simulink model "generic_Truck_And_Trailer"  (R2025a)
settings: Solver=VariableStepAuto  StartTime=0.0  StopTime=350  FixedStep=0.01  MaxStep=0.001  RelTol=1e-3  EnableMultiTasking=on
libraries: TruckMaker4SL x250, simulink x1
(part 4 of 11)

== system generic_Truck_And_Trailer/TruckMaker/Tractor_Subsystem /Subsystem_Noisey Measurements/Measurements from IMU ==
  Acc_x : TruckMaker4SL/Read CM Dict  xname=Sensor.Inertial.Vhcl.VchBdy.Acc_B.x  xsync=off  xstime=Continuous
      settings: SourceProductName=TruckMaker4SL
  Acc_y : TruckMaker4SL/Read CM Dict  xname=Sensor.Inertial.Vhcl.VchBdy.Acc_B.y  xsync=off  xstime=Continuous
      settings: SourceProductName=TruckMaker4SL
  Acc_z : TruckMaker4SL/Read CM Dict  xname=Sensor.Inertial.Vhcl.VchBdy.Acc_B.z  xsync=off  xstime=Continuous
      settings: SourceProductName=TruckMaker4SL
  Omega_z : TruckMaker4SL/Read CM Dict  xname=Sensor.Inertial.Vhcl.VchBdy.Omega_B.z  xsync=off  xstime=Continuous
      settings: SourceProductName=TruckMaker4SL
  Omega_z1 : TruckMaker4SL/Read CM Dict  xname=Sensor.Inertial.Vhcl.VchBdy.Omega_B.y  xsync=off  xstime=Continuous
      settings: SourceProductName=TruckMaker4SL
  Omega_z2 : TruckMaker4SL/Read CM Dict  xname=Sensor.Inertial.Vhcl.VchBdy.Omega_B.x  xsync=off  xstime=Continuous
      settings: SourceProductName=TruckMaker4SL
  Vel_x : TruckMaker4SL/Read CM Dict  xname=Sensor.Inertial.Vhcl.VchBdy.Vel_B.x  xsync=off  xstime=Continuous
      settings: SourceProductName=TruckMaker4SL
  Vel_y : TruckMaker4SL/Read CM Dict  xname=Sensor.Inertial.Vhcl.VchBdy.Vel_B.y  xsync=off  xstime=Continuous
      settings: SourceProductName=TruckMaker4SL
  Vel_z : TruckMaker4SL/Read CM Dict  xname=Sensor.Inertial.Vhcl.VchBdy.Vel_B.z  xsync=off  xstime=Continuous
      settings: SourceProductName=TruckMaker4SL
  acc_x : Outport
  acc_y : Outport  Port=2
  acc_z : Outport  Port=3
  vel_x : Outport  Port=4
  vel_y : Outport  Port=5
  vel_z : Outport  Port=6
  wx : Outport  Port=7
  wy : Outport  Port=8
  wz : Outport  Port=9
  wires:
  Omega_z/1 -> wz/1
  Omega_z1/1 -> wy/1
  Omega_z2/1 -> wx/1
  Vel_z/1 -> vel_z/1
  Vel_y/1 -> vel_y/1
  Vel_x/1 -> vel_x/1
  Acc_z/1 -> acc_z/1
  Acc_y/1 -> acc_y/1
  Acc_x/1 -> acc_x/1

== system generic_Truck_And_Trailer/TruckMaker/Tractor_Subsystem /Subsystem_Noisey Measurements _NAN/Measurements from IMU ==
  Acc_x : TruckMaker4SL/Read CM Dict  xname=Sensor.Inertial.Vhcl.VchBdy.Acc_B.x  xsync=off  xstime=Continuous
      settings: SourceProductName=TruckMaker4SL
  Acc_y : TruckMaker4SL/Read CM Dict  xname=Sensor.Inertial.Vhcl.VchBdy.Acc_B.y  xsync=off  xstime=Continuous
      settings: SourceProductName=TruckMaker4SL
  Acc_z : TruckMaker4SL/Read CM Dict  xname=Sensor.Inertial.Vhcl.VchBdy.Acc_B.z  xsync=off  xstime=Continuous
      settings: SourceProductName=TruckMaker4SL
  Omega_z : TruckMaker4SL/Read CM Dict  xname=Sensor.Inertial.Vhcl.VchBdy.Omega_B.z  xsync=off  xstime=Continuous
      settings: SourceProductName=TruckMaker4SL
  Omega_z1 : TruckMaker4SL/Read CM Dict  xname=Sensor.Inertial.Vhcl.VchBdy.Omega_B.y  xsync=off  xstime=Continuous
      settings: SourceProductName=TruckMaker4SL
  Omega_z2 : TruckMaker4SL/Read CM Dict  xname=Sensor.Inertial.Vhcl.VchBdy.Omega_B.x  xsync=off  xstime=Continuous
      settings: SourceProductName=TruckMaker4SL
  Vel_x : TruckMaker4SL/Read CM Dict  xname=Sensor.Inertial.Vhcl.VchBdy.Vel_B.x  xsync=off  xstime=Continuous
      settings: SourceProductName=TruckMaker4SL
  Vel_y : TruckMaker4SL/Read CM Dict  xname=Sensor.Inertial.Vhcl.VchBdy.Vel_B.y  xsync=off  xstime=Continuous
      settings: SourceProductName=TruckMaker4SL
  Vel_z : TruckMaker4SL/Read CM Dict  xname=Sensor.Inertial.Vhcl.VchBdy.Vel_B.z  xsync=off  xstime=Continuous
      settings: SourceProductName=TruckMaker4SL
  acc_x : Outport
  acc_y : Outport  Port=2
  acc_z : Outport  Port=3
  vel_x : Outport  Port=4
  vel_y : Outport  Port=5
  vel_z : Outport  Port=6
  wx : Outport  Port=7
  wy : Outport  Port=8
  wz : Outport  Port=9
  wires:
  Acc_x/1 -> acc_x/1
  Acc_y/1 -> acc_y/1
  Acc_z/1 -> acc_z/1
  Vel_x/1 -> vel_x/1
  Vel_y/1 -> vel_y/1
  Vel_z/1 -> vel_z/1
  Omega_z2/1 -> wx/1
  Omega_z1/1 -> wy/1
  Omega_z/1 -> wz/1

== system generic_Truck_And_Trailer/TruckMaker/IPG Vehicle/CarAndTrailer/CarAndTrailerUpd/CreateBus Brake.IF.In ==
  In : Inport
  BusCreator : BusCreator  Inputs=25
  Demux : Demux  Outputs=25
      settings: DisplayOption=none
  Out : Outport  VectorParamsAs1DForOutWhenUnconnected=off
  wires:
  Demux/25 -> BusCreator/25  "Brake IF Trq_Reg RR4"
  Demux/24 -> BusCreator/24  "Brake IF Trq_Reg RL4"
  Demux/23 -> BusCreator/23  "Brake IF Trq_Reg RR3"
  Demux/22 -> BusCreator/22  "Brake IF Trq_Reg RL3"
  Demux/21 -> BusCreator/21  "Brake IF Trq_Reg FR2"
  Demux/20 -> BusCreator/20  "Brake IF Trq_Reg FL2"
  Demux/19 -> BusCreator/19  "Brake IF Trq_Reg RR2"
  Demux/18 -> BusCreator/18  "Brake IF Trq_Reg RL2"
  Demux/17 -> BusCreator/17  "Brake IF Trq_Reg RR"
  Demux/16 -> BusCreator/16  "Brake IF Trq_Reg RL"
  Demux/15 -> BusCreator/15  "Brake IF Trq_Reg FR"
  Demux/14 -> BusCreator/14  "Brake IF Trq_Reg FL"
  Demux/13 -> BusCreator/13  "Brake IF Trq_Reg_max RR4"
  Demux/12 -> BusCreator/12  "Brake IF Trq_Reg_max RL4"
  Demux/11 -> BusCreator/11  "Brake IF Trq_Reg_max RR3"
  Demux/10 -> BusCreator/10  "Brake IF Trq_Reg_max RL3"
  Demux/9 -> BusCreator/9  "Brake IF Trq_Reg_max FR2"
  Demux/8 -> BusCreator/8  "Brake IF Trq_Reg_max FL2"
  Demux/7 -> BusCreator/7  "Brake IF Trq_Reg_max RR2"
  Demux/6 -> BusCreator/6  "Brake IF Trq_Reg_max RL2"
  Demux/5 -> BusCreator/5  "Brake IF Trq_Reg_max RR"
  Demux/4 -> BusCreator/4  "Brake IF Trq_Reg_max RL"
  Demux/3 -> BusCreator/3  "Brake IF Trq_Reg_max FR"
  Demux/2 -> BusCreator/2  "Brake IF Trq_Reg_max FL"
  Demux/1 -> BusCreator/1  "Brake IF T_env"
  BusCreator/1 -> Out/1
  In/1 -> Demux/1

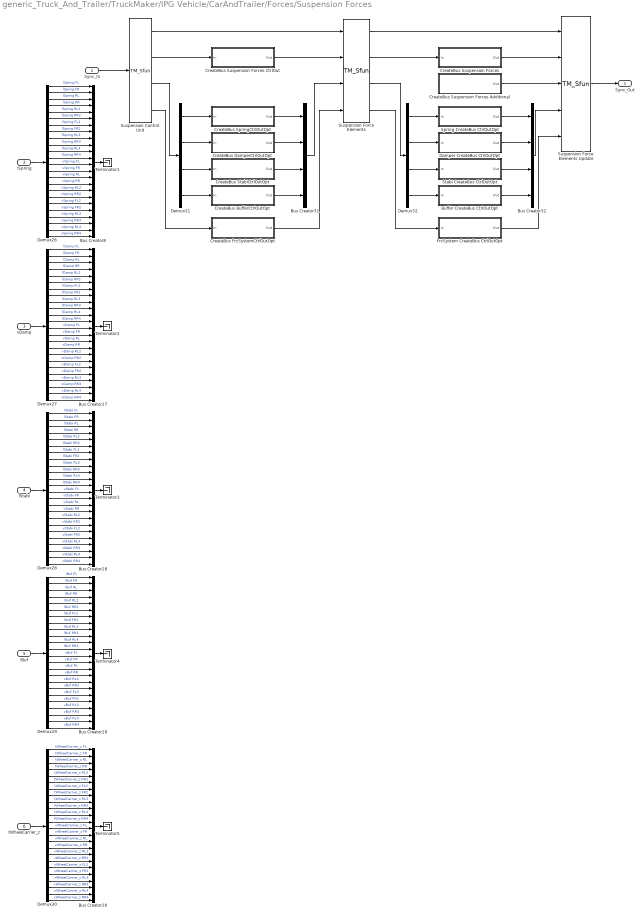
== system generic_Truck_And_Trailer/TruckMaker/IPG Vehicle/CarAndTrailer/Forces/Suspension Forces ==
  Sync_In : Inport
  lSpring : Inport  Port=2
  vDamp : Inport  Port=3
  lStabi : Inport  Port=4
  lBuf : Inport  Port=5
  tWheelCarrier_z : Inport  Port=6
  Buffer CreateBus CtrlOutOpt : Subsystem
  Bus Creator{8,27..30} (5 alike) : BusCreator  Inputs=24
  Bus Creator31 : BusCreator  Inputs=4
  Bus Creator32 : BusCreator  Inputs=4
  CreateBus BufferCtrlOutOpt : Subsystem
  CreateBus DamperCtrlOutOpt : Subsystem
  CreateBus FrcSystemCtrlOutOpt : Subsystem
  CreateBus SpringCtrlOutOpt : Subsystem
  CreateBus StabiCtrlOutOpt : Subsystem
  CreateBus Suspension Forces : Subsystem
  CreateBus Suspension Forces Additional : Subsystem
  CreateBus Suspension Forces CtrlOut : Subsystem
  Damper CreateBus CtrlOutOpt : Subsystem
  Demux{26..30} (5 alike) : Demux  Outputs=24
      settings: DisplayOption=none
  Demux31 : Demux
      settings: DisplayOption=none
  Demux32 : Demux
      settings: DisplayOption=none
  FrcSystem CreateBus CtrlOutOpt : Subsystem
  Spring CreateBus CtrlOutOpt : Subsystem
  Stabi CreateBus CtrlOutOpt : Subsystem
  Suspension Control Unit : S-Function  FunctionName=TM_Sfun  Parameters='ForcesSuspControl'  SFunctionDeploymentMode=off  EnableBusSupport=off
  Suspension Force Elements : S-Function  FunctionName=TM_Sfun  Parameters='ForcesSusp'  SFunctionDeploymentMode=off  EnableBusSupport=off
  Suspension Force Elements Update : S-Function  FunctionName=TM_Sfun  Parameters='ForcesSuspUpd'  SFunctionDeploymentMode=off  EnableBusSupport=off
  Terminator{1..5} (5 alike) : Terminator
  Sync_Out : Outport  VectorParamsAs1DForOutWhenUnconnected=off
  wires:
  CreateBus Suspension Forces CtrlOut/1(Out) -> Suspension Force Elements/2
  Suspension Control Unit/2 -> CreateBus Suspension Forces CtrlOut/1(In)
  Suspension Force Elements Update/1 -> Sync_Out/1
  Suspension Force Elements/1 -> Suspension Force Elements Update/1
  Suspension Control Unit/1 -> Suspension Force Elements/1
  Sync_In/1 -> Suspension Control Unit/1
  CreateBus Suspension Forces Additional/1(Out) -> Suspension Force Elements Update/3
  Demux27/20 -> Bus Creator27/20  "vDamp FR2"
  Demux29/8 -> Bus Creator29/8  "lBuf FR2"
  Demux27/10 -> Bus Creator27/10  "lDamp RR3"
  Demux29/12 -> Bus Creator29/12  "lBuf RR4"
  Demux26/21 -> Bus Creator8/21  "vSpring RL3"
  Demux29/11 -> Bus Creator29/11  "lBuf RL4"
  Demux26/5 -> Bus Creator8/5  "lSpring RL2"
  Demux27/23 -> Bus Creator27/23  "vDamp RL4"
  Demux27/7 -> Bus Creator27/7  "lDamp FL2"
  Demux29/17 -> Bus Creator29/17  "vBuf RL2"
  lBuf/1 -> Demux29/1
  Demux27/21 -> Bus Creator27/21  "vDamp RL3"
  Demux26/17 -> Bus Creator8/17  "vSpring RL2"
  Demux28/17 -> Bus Creator28/17  "vStabi RL2"
  Demux27/6 -> Bus Creator27/6  "lDamp RR2"
  Demux26/16 -> Bus Creator8/16  "vSpring RR"
  vDamp/1 -> Demux27/1
  Demux28/13 -> Bus Creator28/13  "vStabi FL"
  Demux27/3 -> Bus Creator27/3  "lDamp RL"
  Demux28/24 -> Bus Creator28/24  "vStabi RR4"
  Demux29/9 -> Bus Creator29/9  "lBuf RL3"
  Demux27/17 -> Bus Creator27/17  "vDamp RL2"
  Demux28/9 -> Bus Creator28/9  "lStabi RL3"
  Demux29/5 -> Bus Creator29/5  "lBuf RL2"
  Demux28/12 -> Bus Creator28/12  "lStabi RR4"
  Demux26/12 -> Bus Creator8/12  "lSpring RR4"
  Demux26/24 -> Bus Creator8/24  "vSpring RR4"
  Demux28/23 -> Bus Creator28/23  "vStabi RL4"
  Demux26/4 -> Bus Creator8/4  "lSpring RR"
  Demux28/4 -> Bus Creator28/4  "lStabi RR"
  Demux29/3 -> Bus Creator29/3  "lBuf RL"
  Demux28/14 -> Bus Creator28/14  "vStabi FR"
  Demux27/12 -> Bus Creator27/12  "lDamp RR4"
  Demux28/8 -> Bus Creator28/8  "lStabi FR2"
  Demux29/6 -> Bus Creator29/6  "lBuf RR2"
  Demux27/14 -> Bus Creator27/14  "vDamp FR"
  Bus Creator29/1 -> Terminator4/1
  Demux28/7 -> Bus Creator28/7  "lStabi FL2"
  Demux29/1 -> Bus Creator29/1  "lBuf FL"
  Demux27/2 -> Bus Creator27/2  "lDamp FR"
  Demux26/9 -> Bus Creator8/9  "lSpring RL3"
  Demux26/7 -> Bus Creator8/7  "lSpring FL2"
  Demux29/4 -> Bus Creator29/4  "lBuf RR"
  Demux28/11 -> Bus Creator28/11  "lStabi RL4"
  Demux28/10 -> Bus Creator28/10  "lStabi RR3"
  Demux28/1 -> Bus Creator28/1  "lStabi FL"
  lStabi/1 -> Demux28/1
  Demux26/14 -> Bus Creator8/14  "vSpring FR"
  Demux28/21 -> Bus Creator28/21  "vStabi RL3"
  Demux26/15 -> Bus Creator8/15  "vSpring RL"
  Demux28/2 -> Bus Creator28/2  "lStabi FR"
  Demux28/15 -> Bus Creator28/15  "vStabi RL"
  Demux28/19 -> Bus Creator28/19  "vStabi FL2"
  Demux28/16 -> Bus Creator28/16  "vStabi RR"
  Demux28/6 -> Bus Creator28/6  "lStabi RR2"
  Demux29/22 -> Bus Creator29/22  "vBuf RR3"
  Demux27/15 -> Bus Creator27/15  "vDamp RL"
  Demux27/5 -> Bus Creator27/5  "lDamp RL2"
  Demux29/15 -> Bus Creator29/15  "vBuf RL"
  Demux29/13 -> Bus Creator29/13  "vBuf FL"
  Demux26/13 -> Bus Creator8/13  "vSpring FL"
  Demux27/1 -> Bus Creator27/1  "lDamp FL"
  Demux26/18 -> Bus Creator8/18  "vSpring RR2"
  Demux28/5 -> Bus Creator28/5  "lStabi RL2"
  Demux29/10 -> Bus Creator29/10  "lBuf RR3"
  Demux28/18 -> Bus Creator28/18  "vStabi RR2"
  Demux27/11 -> Bus Creator27/11  "lDamp RL4"
  Demux27/9 -> Bus Creator27/9  "lDamp RL3"
  Demux27/18 -> Bus Creator27/18  "vDamp RR2"
  Demux29/16 -> Bus Creator29/16  "vBuf RR"
  Demux27/8 -> Bus Creator27/8  "lDamp FR2"
  Demux26/2 -> Bus Creator8/2  "lSpring FR"
  Demux26/1 -> Bus Creator8/1  "lSpring FL"
  Demux29/24 -> Bus Creator29/24  "vBuf RR4"
  Demux27/19 -> Bus Creator27/19  "vDamp FL2"
  Demux29/2 -> Bus Creator29/2  "lBuf FR"
  Demux27/24 -> Bus Creator27/24  "vDamp RR4"
  Demux27/4 -> Bus Creator27/4  "lDamp RR"
  Demux26/3 -> Bus Creator8/3  "lSpring RL"
  Demux28/20 -> Bus Creator28/20  "vStabi FR2"
  Demux26/6 -> Bus Creator8/6  "lSpring RR2"
  Demux29/14 -> Bus Creator29/14  "vBuf FR"
  Demux27/16 -> Bus Creator27/16  "vDamp RR"
  Demux27/22 -> Bus Creator27/22  "vDamp RR3"
  lSpring/1 -> Demux26/1
  Demux26/11 -> Bus Creator8/11  "lSpring RL4"
  Demux26/22 -> Bus Creator8/22  "vSpring RR3"
  Bus Creator27/1 -> Terminator2/1
  Demux29/18 -> Bus Creator29/18  "vBuf RR2"
  Demux26/10 -> Bus Creator8/10  "lSpring RR3"
  Bus Creator28/1 -> Terminator3/1
  Demux26/8 -> Bus Creator8/8  "lSpring FR2"
  Demux26/19 -> Bus Creator8/19  "vSpring FL2"
  Bus Creator8/1 -> Terminator1/1
  Demux29/23 -> Bus Creator29/23  "vBuf RL4"
  Demux29/21 -> Bus Creator29/21  "vBuf RL3"
  Demux26/23 -> Bus Creator8/23  "vSpring RL4"
  Demux29/19 -> Bus Creator29/19  "vBuf FL2"
  Demux28/22 -> Bus Creator28/22  "vStabi RR3"
  Demux28/3 -> Bus Creator28/3  "lStabi RL"
  Demux27/13 -> Bus Creator27/13  "vDamp FL"
  Demux29/7 -> Bus Creator29/7  "lBuf FL2"
  Demux26/20 -> Bus Creator8/20  "vSpring FR2"
  Demux29/20 -> Bus Creator29/20  "vBuf FR2"
  Demux30/15 -> Bus Creator30/15  "vWheelCarrier_z RL"
  Demux30/11 -> Bus Creator30/11  "tWheelCarrier_z RL4"
  Demux30/16 -> Bus Creator30/16  "vWheelCarrier_z RR"
  Demux30/24 -> Bus Creator30/24  "vWheelCarrier_z RR4"
  Demux30/8 -> Bus Creator30/8  "tWheelCarrier_z FR2"
  Demux30/18 -> Bus Creator30/18  "vWheelCarrier_z RR2"
  Demux30/9 -> Bus Creator30/9  "tWheelCarrier_z RL3"
  Demux30/22 -> Bus Creator30/22  "vWheelCarrier_z RR3"
  Demux30/3 -> Bus Creator30/3  "tWheelCarrier_z RL"
  Bus Creator30/1 -> Terminator5/1
  Demux30/7 -> Bus Creator30/7  "tWheelCarrier_z FL2"
  Demux30/5 -> Bus Creator30/5  "tWheelCarrier_z RL2"
  Demux30/21 -> Bus Creator30/21  "vWheelCarrier_z RL3"
  Demux30/10 -> Bus Creator30/10  "tWheelCarrier_z RR3"
  Demux30/2 -> Bus Creator30/2  "tWheelCarrier_z FR"
  Demux30/19 -> Bus Creator30/19  "vWheelCarrier_z FL2"
  Demux30/4 -> Bus Creator30/4  "tWheelCarrier_z RR"
  Demux30/23 -> Bus Creator30/23  "vWheelCarrier_z RL4"
  Demux30/13 -> Bus Creator30/13  "vWheelCarrier_z FL"
  Demux30/17 -> Bus Creator30/17  "vWheelCarrier_z RL2"
  Demux30/14 -> Bus Creator30/14  "vWheelCarrier_z FR"
  Demux30/6 -> Bus Creator30/6  "tWheelCarrier_z RR2"
  Demux30/20 -> Bus Creator30/20  "vWheelCarrier_z FR2"
  tWheelCarrier_z/1 -> Demux30/1
  Demux30/12 -> Bus Creator30/12  "tWheelCarrier_z RR4"
  Demux30/1 -> Bus Creator30/1  "tWheelCarrier_z FL"
  CreateBus DamperCtrlOutOpt/1(Out) -> Bus Creator31/2
  CreateBus StabiCtrlOutOpt/1(Out) -> Bus Creator31/3
  Suspension Control Unit/4 -> CreateBus FrcSystemCtrlOutOpt/1(In)
  CreateBus SpringCtrlOutOpt/1(Out) -> Bus Creator31/1
  Demux31/3 -> CreateBus StabiCtrlOutOpt/1(In)
  Demux31/2 -> CreateBus DamperCtrlOutOpt/1(In)
  Demux31/1 -> CreateBus SpringCtrlOutOpt/1(In)
  CreateBus FrcSystemCtrlOutOpt/1(Out) -> Suspension Force Elements/4
  Demux31/4 -> CreateBus BufferCtrlOutOpt/1(In)
  CreateBus BufferCtrlOutOpt/1(Out) -> Bus Creator31/4
  Suspension Control Unit/3 -> Demux31/1
  Bus Creator31/1 -> Suspension Force Elements/3
  Spring CreateBus CtrlOutOpt/1(Out) -> Bus Creator32/1
  Demux32/2 -> Damper CreateBus CtrlOutOpt/1(In)
  Damper CreateBus CtrlOutOpt/1(Out) -> Bus Creator32/2
  Buffer CreateBus CtrlOutOpt/1(Out) -> Bus Creator32/4
  Demux32/4 -> Buffer CreateBus CtrlOutOpt/1(In)
  Demux32/1 -> Spring CreateBus CtrlOutOpt/1(In)
  Stabi CreateBus CtrlOutOpt/1(Out) -> Bus Creator32/3
  Demux32/3 -> Stabi CreateBus CtrlOutOpt/1(In)
  Suspension Force Elements/2 -> CreateBus Suspension Forces/1(In)
  CreateBus Suspension Forces/1(Out) -> Suspension Force Elements Update/2
  Suspension Force Elements/3 -> Demux32/1
  Suspension Force Elements/4 -> FrcSystem CreateBus CtrlOutOpt/1(In)
  Bus Creator32/1 -> Suspension Force Elements Update/4
  FrcSystem CreateBus CtrlOutOpt/1(Out) -> Suspension Force Elements Update/5

== system generic_Truck_And_Trailer/TruckMaker/IPG Vehicle/CarAndTrailer/Forces/Vehicle Forces ==
  Sync_In : Inport
  Bus Creator1 : BusCreator  Inputs=12
  Bus Creator8 : BusCreator  Inputs=16
  BusCreator1 : BusCreator  Inputs=4
  BusCreator2 : BusCreator  Inputs=9
  Demux : Demux  Outputs=16
      settings: DisplayOption=none
  Demux1 : Demux  Outputs=12
      settings: DisplayOption=none
  Demux2 : Demux  Outputs=13
      settings: DisplayOption=none
  Forces : S-Function  FunctionName=TM_Sfun  Parameters='Forces'  SFunctionDeploymentMode=off  EnableBusSupport=off
  Terminator : Terminator
  Sync_Out : Outport  VectorParamsAs1DForOutWhenUnconnected=off
  Car.Virtual : Outport  Port=2  VectorParamsAs1DForOutWhenUnconnected=off
  Car.Aero : Outport  Port=3  VectorParamsAs1DForOutWhenUnconnected=off
  Car.Load : Outport  Port=4  VectorParamsAs1DForOutWhenUnconnected=off
  wires:
  BusCreator1/1 -> Terminator/1  "Aero IF (in)"
  Demux2/13 -> BusCreator2/9  "car Aero Trq_1 z"
  Demux2/12 -> BusCreator2/8  "car Aero Trq_1 y"
  Demux2/11 -> BusCreator2/7  "car Aero Trq_1 x"
  Demux2/10 -> BusCreator2/6  "car Aero Frc_1 z"
  Demux2/9 -> BusCreator2/5  "car Aero Frc_1 y"
  Demux2/8 -> BusCreator2/4  "car Aero Frc_1 x"
  Demux2/7 -> BusCreator2/3  "car Aero PoA_1 z"
  Demux2/6 -> BusCreator2/2  "car Aero PoA_1 y"
  Demux2/5 -> BusCreator2/1  "car Aero PoA_1 x"
  Demux2/4 -> BusCreator1/4  "car Aero tau_1"
  Demux2/3 -> BusCreator1/3  "car Aero ApproachVel_1 z"
  Demux2/2 -> BusCreator1/2  "car Aero ApproachVel_1 y"
  Demux2/1 -> BusCreator1/1  "car Aero ApproachVel_1 x"
  BusCreator2/1 -> Car.Aero/1
  Demux/16 -> Bus Creator8/16  "Car Load_3 tz"
  Demux/15 -> Bus Creator8/15  "Car Load_3 ty"
  Demux/14 -> Bus Creator8/14  "Car Load_3 tx"
  Demux/13 -> Bus Creator8/13  "Car Load_3 mass"
  Demux1/12 -> Bus Creator1/12  "Car Virtual Trq_0 z"
  Demux1/11 -> Bus Creator1/11  "Car Virtual Trq_0 y"
  Demux1/10 -> Bus Creator1/10  "Car Virtual Trq_0 x"
  Demux1/9 -> Bus Creator1/9  "Car Virtual Trq_1 z"
  Demux1/8 -> Bus Creator1/8  "Car Virtual Trq_1 y"
  Demux1/7 -> Bus Creator1/7  "Car Virtual Trq_1 x"
  Demux1/6 -> Bus Creator1/6  "Car Virtual Frc_0 z"
  Demux1/5 -> Bus Creator1/5  "Car Virtual Frc_0 y"
  Demux1/4 -> Bus Creator1/4  "Car Virtual Frc_0 x"
  Sync_In/1 -> Forces/1
  Forces/1 -> Sync_Out/1
  Demux1/1 -> Bus Creator1/1  "Car Virtual Frc_1 x"
  Demux1/2 -> Bus Creator1/2  "Car Virtual Frc_1 y"
  Demux1/3 -> Bus Creator1/3  "Car Virtual Frc_1 z"
  Forces/3 -> Demux2/1
  Forces/2 -> Demux1/1
  Bus Creator1/1 -> Car.Virtual/1
  Bus Creator8/1 -> Car.Load/1
  Demux/1 -> Bus Creator8/1  "Car Load_0 mass"
  Demux/2 -> Bus Creator8/2  "Car Load_0 tx"
  Demux/3 -> Bus Creator8/3  "Car Load_0 ty"
  Demux/4 -> Bus Creator8/4  "Car Load_0 tz"
  Demux/5 -> Bus Creator8/5  "Car Load_1 mass"
  Demux/6 -> Bus Creator8/6  "Car Load_1 tx"
  Demux/7 -> Bus Creator8/7  "Car Load_1 ty"
  Demux/8 -> Bus Creator8/8  "Car Load_1 tz"
  Demux/9 -> Bus Creator8/9  "Car Load_2 mass"
  Demux/10 -> Bus Creator8/10  "Car Load_2 tx"
  Demux/11 -> Bus Creator8/11  "Car Load_2 ty"
  Demux/12 -> Bus Creator8/12  "Car Load_2 tz"
  Forces/4 -> Demux/1

== system generic_Truck_And_Trailer/TruckMaker/IPG Vehicle/CarAndTrailer/Trailer/CreateBus Car.Hitch.FrcTrq ==
  In1 : Inport
  Bus Creator7 : BusCreator  Inputs=6
  Demux7 : Demux  Outputs=6
      settings: DisplayOption=none
  Out1 : Outport  VectorParamsAs1DForOutWhenUnconnected=off
  wires:
  In1/1 -> Demux7/1
  Bus Creator7/1 -> Out1/1
  Demux7/6 -> Bus Creator7/6  "Car Hitch Trq2Car z"
  Demux7/5 -> Bus Creator7/5  "Car Hitch Trq2Car y"
  Demux7/4 -> Bus Creator7/4  "Car Hitch Trq2Car x"
  Demux7/3 -> Bus Creator7/3  "Car Hitch Frc2Car z"
  Demux7/2 -> Bus Creator7/2  "Car Hitch Frc2Car y"
  Demux7/1 -> Bus Creator7/1  "Car Hitch Frc2Car x"

== system generic_Truck_And_Trailer/TruckMaker/IPG Vehicle/CarAndTrailer/Trailer/CreateBus Vhcl.Motion ==
  In1 : Inport
  BusCreator : BusCreator  Inputs=15
  Demux : Demux  Outputs=15
      settings: DisplayOption=none
  Mux : Mux  Inputs=2
  Scope : Scope
      settings: ActiveDisplayYMinimum=-2.4357036031707069  ActiveDisplayYMaximum=21.91421659683628  DataLoggingVariableName=ScopeData2
  Out1 : Outport  VectorParamsAs1DForOutWhenUnconnected=off
  wires:
  Demux/15 -> BusCreator/15  "Vhcl YawAcc"
  Demux/14 -> Mux/2, BusCreator/14  "Vhcl YawVel"
  Demux/13 -> BusCreator/13  "Vhcl Yaw"
  Demux/12 -> BusCreator/12  "Vhcl PitchAcc"
  Demux/11 -> BusCreator/11  "Vhcl PitchVel"
  Demux/10 -> BusCreator/10  "Vhcl Pitch"
  Demux/9 -> BusCreator/9  "Vhcl RollAcc"
  Demux/8 -> BusCreator/8  "Vhcl RollVel"
  Demux/7 -> BusCreator/7  "Vhcl Roll"
  Demux/6 -> BusCreator/6  "Vhcl Hitch_Pos z"
  Demux/5 -> BusCreator/5  "Vhcl Hitch_Pos y"
  Demux/4 -> BusCreator/4  "Vhcl Hitch_Pos x"
  Demux/3 -> BusCreator/3  "Vhcl sRoad"
  Demux/2 -> BusCreator/2  "Vhcl Distance"
  Demux/1 -> Mux/1, BusCreator/1  "Vhcl v"
  In1/1 -> Demux/1
  BusCreator/1 -> Out1/1
  Mux/1 -> Scope/1

== system generic_Truck_And_Trailer/TruckMaker/IPG Vehicle/CarAndTrailer/Trailer/CreateBus Vhcl.PoI ==
  In1 : Inport
  Bus Creator3 : BusCreator  Inputs=18
  Demux3 : Demux  Outputs=18
      settings: DisplayOption=none
  Out1 : Outport  VectorParamsAs1DForOutWhenUnconnected=off
  wires:
  Demux3/18 -> Bus Creator3/18  "Vhcl PoI_GCS Elev"
  Demux3/17 -> Bus Creator3/17  "Vhcl PoI_GCS Lat"
  Demux3/16 -> Bus Creator3/16  "Vhcl PoI_GCS Long"
  Demux3/15 -> Bus Creator3/15  "Vhcl PoI_Acc_1 z"
  Demux3/14 -> Bus Creator3/14  "Vhcl PoI_Acc_1 y"
  Demux3/13 -> Bus Creator3/13  "Vhcl PoI_Acc_1 x"
  Demux3/12 -> Bus Creator3/12  "Vhcl PoI_Vel_1 z"
  Demux3/11 -> Bus Creator3/11  "Vhcl PoI_Vel_1 y"
  Demux3/10 -> Bus Creator3/10  "Vhcl PoI_Vel_1 x"
  Demux3/9 -> Bus Creator3/9  "Vhcl PoI_Acc z"
  Demux3/8 -> Bus Creator3/8  "Vhcl PoI_Acc y"
  Demux3/7 -> Bus Creator3/7  "Vhcl PoI_Acc x"
  Demux3/6 -> Bus Creator3/6  "Vhcl PoI_Vel z"
  Demux3/5 -> Bus Creator3/5  "Vhcl PoI_Vel y"
  Demux3/4 -> Bus Creator3/4  "Vhcl PoI_Vel x"
  Demux3/3 -> Bus Creator3/3  "Vhcl PoI_Pos z"
  Demux3/2 -> Bus Creator3/2  "Vhcl PoI_Pos y"
  In1/1 -> Demux3/1
  Bus Creator3/1 -> Out1/1
  Demux3/1 -> Bus Creator3/1  "Vhcl PoI_Pos x"

== system generic_Truck_And_Trailer/TruckMaker/IPG Vehicle/CarAndTrailer/Trailer/CreateBus Vhcl.Steering ==
  In1 : Inport
  Bus Creator3 : BusCreator  Inputs=4
  Demux : Demux
      settings: DisplayOption=none
  Out1 : Outport  VectorParamsAs1DForOutWhenUnconnected=off
  wires:
  Bus Creator3/1 -> Out1/1
  Demux/1 -> Bus Creator3/1  "Vhcl Steering Ang"
  Demux/3 -> Bus Creator3/3  "Vhcl Steering AngAcc"
  Demux/2 -> Bus Creator3/2  "Vhcl Steering AngVel"
  Demux/4 -> Bus Creator3/4  "Vhcl Steering Trq"
  In1/1 -> Demux/1

== system generic_Truck_And_Trailer/TruckMaker/IPG Vehicle/CarAndTrailer/Trailer/CreateBus Vhcl.Wheel.FL ==
  In1 : Inport
  Bus Creator3 : BusCreator  Inputs=14
  Demux3 : Demux  Outputs=14
      settings: DisplayOption=none
  Out1 : Outport  VectorParamsAs1DForOutWhenUnconnected=off
  wires:
  Demux3/14 -> Bus Creator3/14  "Vhcl Wheel FL Trq_WhlBearing"
  Demux3/13 -> Bus Creator3/13  "Vhcl Wheel FL Trq_T2W"
  Demux3/12 -> Bus Creator3/12  "Vhcl Wheel FL SideSlip"
  Demux3/11 -> Bus Creator3/11  "Vhcl Wheel FL LongSlip"
  Demux3/10 -> Bus Creator3/10  "Vhcl Wheel FL vBelt"
  Demux3/9 -> Bus Creator3/9  "Vhcl Wheel FL Fz"
  Demux3/8 -> Bus Creator3/8  "Vhcl Wheel FL Fy"
  Demux3/7 -> Bus Creator3/7  "Vhcl Wheel FL Fx"
  Demux3/6 -> Bus Creator3/6  "Vhcl Wheel FL r_zxy z"
  Demux3/5 -> Bus Creator3/5  "Vhcl Wheel FL r_zxy y"
  Demux3/4 -> Bus Creator3/4  "Vhcl Wheel FL r_zxy x"
  Demux3/3 -> Bus Creator3/3  "Vhcl Wheel FL t z"
  Demux3/2 -> Bus Creator3/2  "Vhcl Wheel FL t y"
  In1/1 -> Demux3/1
  Bus Creator3/1 -> Out1/1
  Demux3/1 -> Bus Creator3/1  "Vhcl Wheel FL t x"

== system generic_Truck_And_Trailer/TruckMaker/IPG Vehicle/CarAndTrailer/Trailer/CreateBus Vhcl.Wheel.FL2 ==
  In1 : Inport
  Bus Creator3 : BusCreator  Inputs=14
  Demux3 : Demux  Outputs=14
      settings: DisplayOption=none
  Out1 : Outport  VectorParamsAs1DForOutWhenUnconnected=off
  wires:
  Demux3/14 -> Bus Creator3/14  "Vhcl Wheel FL2 Trq_WhlBearing"
  Demux3/13 -> Bus Creator3/13  "Vhcl Wheel FL2 Trq_T2W"
  Demux3/12 -> Bus Creator3/12  "Vhcl Wheel FL2 SideSlip"
  Demux3/11 -> Bus Creator3/11  "Vhcl Wheel FL2 LongSlip"
  Demux3/10 -> Bus Creator3/10  "Vhcl Wheel FL2 vBelt"
  Demux3/9 -> Bus Creator3/9  "Vhcl Wheel FL2 Fz"
  Demux3/8 -> Bus Creator3/8  "Vhcl Wheel FL2 Fy"
  Demux3/7 -> Bus Creator3/7  "Vhcl Wheel FL2 Fx"
  Demux3/6 -> Bus Creator3/6  "Vhcl Wheel FL2 r_zxy z"
  Demux3/5 -> Bus Creator3/5  "Vhcl Wheel FL2 r_zxy y"
  Demux3/4 -> Bus Creator3/4  "Vhcl Wheel FL2 r_zxy x"
  Demux3/3 -> Bus Creator3/3  "Vhcl Wheel FL2 t z"
  Demux3/2 -> Bus Creator3/2  "Vhcl Wheel FL2 t y"
  In1/1 -> Demux3/1
  Bus Creator3/1 -> Out1/1
  Demux3/1 -> Bus Creator3/1  "Vhcl Wheel FL2 t x"

== system generic_Truck_And_Trailer/TruckMaker/IPG Vehicle/CarAndTrailer/Trailer/CreateBus Vhcl.Wheel.FR ==
  In1 : Inport
  Bus Creator3 : BusCreator  Inputs=14
  Demux3 : Demux  Outputs=14
      settings: DisplayOption=none
  Out1 : Outport  VectorParamsAs1DForOutWhenUnconnected=off
  wires:
  Demux3/14 -> Bus Creator3/14  "Vhcl Wheel FR Trq_WhlBearing"
  Demux3/13 -> Bus Creator3/13  "Vhcl Wheel FR Trq_T2W"
  Demux3/12 -> Bus Creator3/12  "Vhcl Wheel FR SideSlip"
  Demux3/11 -> Bus Creator3/11  "Vhcl Wheel FR LongSlip"
  Demux3/10 -> Bus Creator3/10  "Vhcl Wheel FR vBelt"
  Demux3/9 -> Bus Creator3/9  "Vhcl Wheel FR Fz"
  Demux3/8 -> Bus Creator3/8  "Vhcl Wheel FR Fy"
  Demux3/7 -> Bus Creator3/7  "Vhcl Wheel FR Fx"
  Demux3/6 -> Bus Creator3/6  "Vhcl Wheel FR r_zxy z"
  Demux3/5 -> Bus Creator3/5  "Vhcl Wheel FR r_zxy y"
  Demux3/4 -> Bus Creator3/4  "Vhcl Wheel FR r_zxy x"
  Demux3/3 -> Bus Creator3/3  "Vhcl Wheel FR t z"
  Demux3/2 -> Bus Creator3/2  "Vhcl Wheel FR t y"
  In1/1 -> Demux3/1
  Bus Creator3/1 -> Out1/1
  Demux3/1 -> Bus Creator3/1  "Vhcl Wheel FR t x"

== system generic_Truck_And_Trailer/TruckMaker/IPG Vehicle/CarAndTrailer/Trailer/CreateBus Vhcl.Wheel.FR2 ==
  In1 : Inport
  Bus Creator3 : BusCreator  Inputs=14
  Demux3 : Demux  Outputs=14
      settings: DisplayOption=none
  Out1 : Outport  VectorParamsAs1DForOutWhenUnconnected=off
  wires:
  Demux3/14 -> Bus Creator3/14  "Vhcl Wheel FR2 Trq_WhlBearing"
  Demux3/13 -> Bus Creator3/13  "Vhcl Wheel FR2 Trq_T2W"
  Demux3/12 -> Bus Creator3/12  "Vhcl Wheel FR2 SideSlip"
  Demux3/11 -> Bus Creator3/11  "Vhcl Wheel FR2 LongSlip"
  Demux3/10 -> Bus Creator3/10  "Vhcl Wheel FR2 vBelt"
  Demux3/9 -> Bus Creator3/9  "Vhcl Wheel FR2 Fz"
  Demux3/8 -> Bus Creator3/8  "Vhcl Wheel FR2 Fy"
  Demux3/7 -> Bus Creator3/7  "Vhcl Wheel FR2 Fx"
  Demux3/6 -> Bus Creator3/6  "Vhcl Wheel FR2 r_zxy z"
  Demux3/5 -> Bus Creator3/5  "Vhcl Wheel FR2 r_zxy y"
  Demux3/4 -> Bus Creator3/4  "Vhcl Wheel FR2 r_zxy x"
  Demux3/3 -> Bus Creator3/3  "Vhcl Wheel FR2 t z"
  Demux3/2 -> Bus Creator3/2  "Vhcl Wheel FR2 t y"
  In1/1 -> Demux3/1
  Bus Creator3/1 -> Out1/1
  Demux3/1 -> Bus Creator3/1  "Vhcl Wheel FR2 t x"

== system generic_Truck_And_Trailer/TruckMaker/IPG Vehicle/CarAndTrailer/Trailer/CreateBus Vhcl.Wheel.RL ==
  In1 : Inport
  Bus Creator3 : BusCreator  Inputs=14
  Demux3 : Demux  Outputs=14
      settings: DisplayOption=none
  Out1 : Outport  VectorParamsAs1DForOutWhenUnconnected=off
  wires:
  Demux3/14 -> Bus Creator3/14  "Vhcl Wheel RL Trq_WhlBearing"
  Demux3/13 -> Bus Creator3/13  "Vhcl Wheel RL Trq_T2W"
  Demux3/12 -> Bus Creator3/12  "Vhcl Wheel RL SideSlip"
  Demux3/11 -> Bus Creator3/11  "Vhcl Wheel RL LongSlip"
  Demux3/10 -> Bus Creator3/10  "Vhcl Wheel RL vBelt"
  Demux3/9 -> Bus Creator3/9  "Vhcl Wheel RL Fz"
  Demux3/8 -> Bus Creator3/8  "Vhcl Wheel RL Fy"
  Demux3/7 -> Bus Creator3/7  "Vhcl Wheel RL Fx"
  Demux3/6 -> Bus Creator3/6  "Vhcl Wheel RL r_zxy z"
  Demux3/5 -> Bus Creator3/5  "Vhcl Wheel RL r_zxy y"
  Demux3/4 -> Bus Creator3/4  "Vhcl Wheel RL r_zxy x"
  Demux3/3 -> Bus Creator3/3  "Vhcl Wheel RL t z"
  Demux3/2 -> Bus Creator3/2  "Vhcl Wheel RL t y"
  In1/1 -> Demux3/1
  Bus Creator3/1 -> Out1/1
  Demux3/1 -> Bus Creator3/1  "Vhcl Wheel RL t x"

== system generic_Truck_And_Trailer/TruckMaker/IPG Vehicle/CarAndTrailer/Trailer/CreateBus Vhcl.Wheel.RL2 ==
  In1 : Inport
  Bus Creator3 : BusCreator  Inputs=14
  Demux3 : Demux  Outputs=14
      settings: DisplayOption=none
  Out1 : Outport  VectorParamsAs1DForOutWhenUnconnected=off
  wires:
  Demux3/14 -> Bus Creator3/14  "Vhcl Wheel RL2 Trq_WhlBearing"
  Demux3/13 -> Bus Creator3/13  "Vhcl Wheel RL2 Trq_T2W"
  Demux3/12 -> Bus Creator3/12  "Vhcl Wheel RL2 SideSlip"
  Demux3/11 -> Bus Creator3/11  "Vhcl Wheel RL2 LongSlip"
  Demux3/10 -> Bus Creator3/10  "Vhcl Wheel RL2 vBelt"
  Demux3/9 -> Bus Creator3/9  "Vhcl Wheel RL2 Fz"
  Demux3/8 -> Bus Creator3/8  "Vhcl Wheel RL2 Fy"
  Demux3/7 -> Bus Creator3/7  "Vhcl Wheel RL2 Fx"
  Demux3/6 -> Bus Creator3/6  "Vhcl Wheel RL2 r_zxy z"
  Demux3/5 -> Bus Creator3/5  "Vhcl Wheel RL2 r_zxy y"
  Demux3/4 -> Bus Creator3/4  "Vhcl Wheel RL2 r_zxy x"
  Demux3/3 -> Bus Creator3/3  "Vhcl Wheel RL2 t z"
  Demux3/2 -> Bus Creator3/2  "Vhcl Wheel RL2 t y"
  In1/1 -> Demux3/1
  Bus Creator3/1 -> Out1/1
  Demux3/1 -> Bus Creator3/1  "Vhcl Wheel RL2 t x"

== system generic_Truck_And_Trailer/TruckMaker/IPG Vehicle/CarAndTrailer/Trailer/CreateBus Vhcl.Wheel.RL3 ==
  In1 : Inport
  Bus Creator3 : BusCreator  Inputs=14
  Demux3 : Demux  Outputs=14
      settings: DisplayOption=none
  Out1 : Outport  VectorParamsAs1DForOutWhenUnconnected=off
  wires:
  Demux3/1 -> Bus Creator3/1  "Vhcl Wheel RL3 t x"
  Bus Creator3/1 -> Out1/1
  In1/1 -> Demux3/1
  Demux3/2 -> Bus Creator3/2  "Vhcl Wheel RL3 t y"
  Demux3/3 -> Bus Creator3/3  "Vhcl Wheel RL3 t z"
  Demux3/4 -> Bus Creator3/4  "Vhcl Wheel RL3 r_zxy x"
  Demux3/5 -> Bus Creator3/5  "Vhcl Wheel RL3 r_zxy y"
  Demux3/6 -> Bus Creator3/6  "Vhcl Wheel RL3 r_zxy z"
  Demux3/7 -> Bus Creator3/7  "Vhcl Wheel RL3 Fx"
  Demux3/8 -> Bus Creator3/8  "Vhcl Wheel RL3 Fy"
  Demux3/9 -> Bus Creator3/9  "Vhcl Wheel RL3 Fz"
  Demux3/10 -> Bus Creator3/10  "Vhcl Wheel RL3 vBelt"
  Demux3/11 -> Bus Creator3/11  "Vhcl Wheel RL3 LongSlip"
  Demux3/12 -> Bus Creator3/12  "Vhcl Wheel RL3 SideSlip"
  Demux3/13 -> Bus Creator3/13  "Vhcl Wheel RL3 Trq_T2W"
  Demux3/14 -> Bus Creator3/14  "Vhcl Wheel RL3 Trq_WhlBearing"

== system generic_Truck_And_Trailer/TruckMaker/IPG Vehicle/CarAndTrailer/Trailer/CreateBus Vhcl.Wheel.RL4 ==
  In1 : Inport
  Bus Creator3 : BusCreator  Inputs=14
  Demux3 : Demux  Outputs=14
      settings: DisplayOption=none
  Out1 : Outport  VectorParamsAs1DForOutWhenUnconnected=off
  wires:
  Demux3/14 -> Bus Creator3/14  "Vhcl Wheel RL4 Trq_WhlBearing"
  Demux3/13 -> Bus Creator3/13  "Vhcl Wheel RL4 Trq_T2W"
  Demux3/12 -> Bus Creator3/12  "Vhcl Wheel RL4 SideSlip"
  Demux3/11 -> Bus Creator3/11  "Vhcl Wheel RL4 LongSlip"
  Demux3/10 -> Bus Creator3/10  "Vhcl Wheel RL4 vBelt"
  Demux3/9 -> Bus Creator3/9  "Vhcl Wheel RL4 Fz"
  Demux3/8 -> Bus Creator3/8  "Vhcl Wheel RL4 Fy"
  Demux3/7 -> Bus Creator3/7  "Vhcl Wheel RL4 Fx"
  Demux3/6 -> Bus Creator3/6  "Vhcl Wheel RL4 r_zxy z"
  Demux3/5 -> Bus Creator3/5  "Vhcl Wheel RL4 r_zxy y"
  Demux3/4 -> Bus Creator3/4  "Vhcl Wheel RL4 r_zxy x"
  Demux3/3 -> Bus Creator3/3  "Vhcl Wheel RL4 t z"
  Demux3/2 -> Bus Creator3/2  "Vhcl Wheel RL4 t y"
  In1/1 -> Demux3/1
  Bus Creator3/1 -> Out1/1
  Demux3/1 -> Bus Creator3/1  "Vhcl Wheel RL4 t x"

== system generic_Truck_And_Trailer/TruckMaker/IPG Vehicle/CarAndTrailer/Trailer/CreateBus Vhcl.Wheel.RR ==
  In1 : Inport
  Bus Creator3 : BusCreator  Inputs=14
  Demux3 : Demux  Outputs=14
      settings: DisplayOption=none
  Out1 : Outport  VectorParamsAs1DForOutWhenUnconnected=off
  wires:
  Demux3/14 -> Bus Creator3/14  "Vhcl Wheel RR Trq_WhlBearing"
  Demux3/12 -> Bus Creator3/12  "Vhcl Wheel RR SideSlip"
  Demux3/11 -> Bus Creator3/11  "Vhcl Wheel RR LongSlip"
  Demux3/10 -> Bus Creator3/10  "Vhcl Wheel RR vBelt"
  Demux3/9 -> Bus Creator3/9  "Vhcl Wheel RR Fz"
  Demux3/8 -> Bus Creator3/8  "Vhcl Wheel RR Fy"
  Demux3/7 -> Bus Creator3/7  "Vhcl Wheel RR Fx"
  Demux3/6 -> Bus Creator3/6  "Vhcl Wheel RR r_zxy z"
  Demux3/5 -> Bus Creator3/5  "Vhcl Wheel RR r_zxy y"
  Demux3/4 -> Bus Creator3/4  "Vhcl Wheel RR r_zxy x"
  Demux3/3 -> Bus Creator3/3  "Vhcl Wheel RR t z"
  Demux3/2 -> Bus Creator3/2  "Vhcl Wheel RR t y"
  In1/1 -> Demux3/1
  Bus Creator3/1 -> Out1/1
  Demux3/1 -> Bus Creator3/1  "Vhcl Wheel RR t x"
  Demux3/13 -> Bus Creator3/13  "Vhcl Wheel RR Trq_T2W"

== system generic_Truck_And_Trailer/TruckMaker/IPG Vehicle/CarAndTrailer/Trailer/CreateBus Vhcl.Wheel.RR2 ==
  In1 : Inport
  Bus Creator3 : BusCreator  Inputs=14
  Demux3 : Demux  Outputs=14
      settings: DisplayOption=none
  Out1 : Outport  VectorParamsAs1DForOutWhenUnconnected=off
  wires:
  Demux3/14 -> Bus Creator3/14  "Vhcl Wheel RR2 Trq_WhlBearing"
  Demux3/13 -> Bus Creator3/13  "Vhcl Wheel RR2 Trq_T2W"
  Demux3/12 -> Bus Creator3/12  "Vhcl Wheel RR2 SideSlip"
  Demux3/11 -> Bus Creator3/11  "Vhcl Wheel RR2 LongSlip"
  Demux3/10 -> Bus Creator3/10  "Vhcl Wheel RR2 vBelt"
  Demux3/9 -> Bus Creator3/9  "Vhcl Wheel RR2 Fz"
  Demux3/8 -> Bus Creator3/8  "Vhcl Wheel RR2 Fy"
  Demux3/7 -> Bus Creator3/7  "Vhcl Wheel RR2 Fx"
  Demux3/6 -> Bus Creator3/6  "Vhcl Wheel RR2 r_zxy z"
  Demux3/5 -> Bus Creator3/5  "Vhcl Wheel RR2 r_zxy y"
  Demux3/4 -> Bus Creator3/4  "Vhcl Wheel RR2 r_zxy x"
  Demux3/3 -> Bus Creator3/3  "Vhcl Wheel RR2 t z"
  Demux3/2 -> Bus Creator3/2  "Vhcl Wheel RR2 t y"
  In1/1 -> Demux3/1
  Bus Creator3/1 -> Out1/1
  Demux3/1 -> Bus Creator3/1  "Vhcl Wheel RR2 t x"

== system generic_Truck_And_Trailer/TruckMaker/IPG Vehicle/CarAndTrailer/Trailer/CreateBus Vhcl.Wheel.RR3 ==
  In1 : Inport
  Bus Creator3 : BusCreator  Inputs=14
  Demux3 : Demux  Outputs=14
      settings: DisplayOption=none
  Out1 : Outport  VectorParamsAs1DForOutWhenUnconnected=off
  wires:
  Demux3/1 -> Bus Creator3/1  "Vhcl Wheel RR3 t x"
  Bus Creator3/1 -> Out1/1
  In1/1 -> Demux3/1
  Demux3/2 -> Bus Creator3/2  "Vhcl Wheel RR3 t y"
  Demux3/3 -> Bus Creator3/3  "Vhcl Wheel RR3 t z"
  Demux3/4 -> Bus Creator3/4  "Vhcl Wheel RR3 r_zxy x"
  Demux3/5 -> Bus Creator3/5  "Vhcl Wheel RR3 r_zxy y"
  Demux3/6 -> Bus Creator3/6  "Vhcl Wheel RR3 r_zxy z"
  Demux3/7 -> Bus Creator3/7  "Vhcl Wheel RR3 Fx"
  Demux3/8 -> Bus Creator3/8  "Vhcl Wheel RR3 Fy"
  Demux3/9 -> Bus Creator3/9  "Vhcl Wheel RR3 Fz"
  Demux3/10 -> Bus Creator3/10  "Vhcl Wheel RR3 vBelt"
  Demux3/11 -> Bus Creator3/11  "Vhcl Wheel RR3 LongSlip"
  Demux3/12 -> Bus Creator3/12  "Vhcl Wheel RR3 SideSlip"
  Demux3/13 -> Bus Creator3/13  "Vhcl Wheel RR3 Trq_T2W"
  Demux3/14 -> Bus Creator3/14  "Vhcl Wheel RR3 Trq_WhlBearing"

== system generic_Truck_And_Trailer/TruckMaker/IPG Vehicle/CarAndTrailer/Trailer/CreateBus Vhcl.Wheel.RR4 ==
  In1 : Inport
  Bus Creator3 : BusCreator  Inputs=14
  Demux3 : Demux  Outputs=14
      settings: DisplayOption=none
  Out1 : Outport  VectorParamsAs1DForOutWhenUnconnected=off
  wires:
  Demux3/14 -> Bus Creator3/14  "Vhcl Wheel RR4 Trq_WhlBearing"
  Demux3/13 -> Bus Creator3/13  "Vhcl Wheel RR4 Trq_T2W"
  Demux3/12 -> Bus Creator3/12  "Vhcl Wheel RR4 SideSlip"
  Demux3/11 -> Bus Creator3/11  "Vhcl Wheel RR4 LongSlip"
  Demux3/10 -> Bus Creator3/10  "Vhcl Wheel RR4 vBelt"
  Demux3/9 -> Bus Creator3/9  "Vhcl Wheel RR4 Fz"
  Demux3/8 -> Bus Creator3/8  "Vhcl Wheel RR4 Fy"
  Demux3/7 -> Bus Creator3/7  "Vhcl Wheel RR4 Fx"
  Demux3/6 -> Bus Creator3/6  "Vhcl Wheel RR4 r_zxy z"
  Demux3/5 -> Bus Creator3/5  "Vhcl Wheel RR4 r_zxy y"
  Demux3/4 -> Bus Creator3/4  "Vhcl Wheel RR4 r_zxy x"
  Demux3/3 -> Bus Creator3/3  "Vhcl Wheel RR4 t z"
  Demux3/2 -> Bus Creator3/2  "Vhcl Wheel RR4 t y"
  In1/1 -> Demux3/1
  Bus Creator3/1 -> Out1/1
  Demux3/1 -> Bus Creator3/1  "Vhcl Wheel RR4 t x"

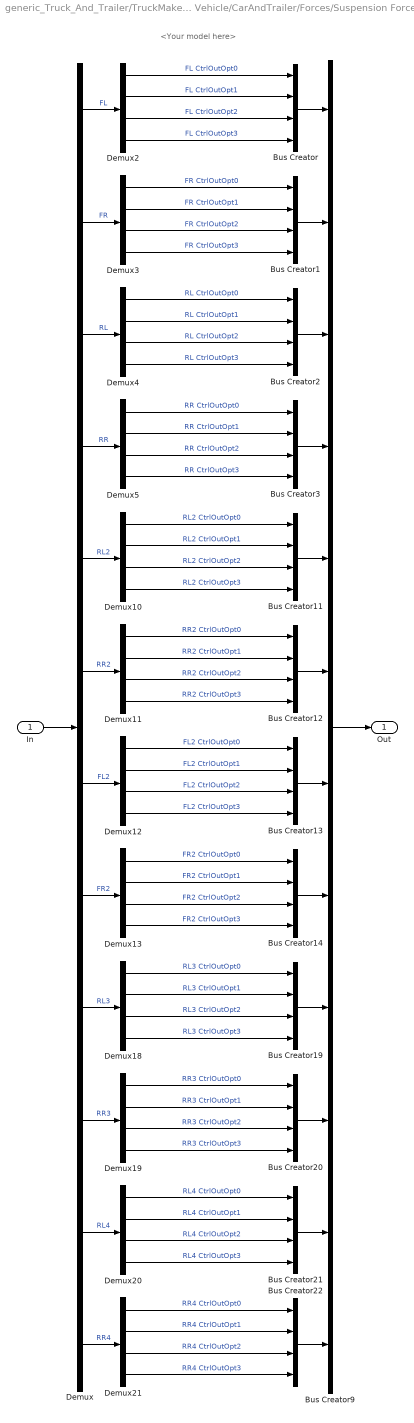
== system generic_Truck_And_Trailer/TruckMaker/IPG Vehicle/CarAndTrailer/Forces/Suspension Forces/Buffer CreateBus CtrlOutOpt ==
  note: <Your model here>
  In : Inport
  Bus Creator{,1..3,11..14,19..22} (12 alike) : BusCreator  Inputs=4
  Bus Creator9 : BusCreator  Inputs=12
  Demux : Demux  Outputs=12
  Demux{2..5,10..13,18..21} (12 alike) : Demux
  Out : Outport
  wires:
  Demux/8 -> Demux13/1  "FR2"
  Demux19/1 -> Bus Creator20/1  "RR3 CtrlOutOpt0"
  Demux19/3 -> Bus Creator20/3  "RR3 CtrlOutOpt2"
  Demux18/4 -> Bus Creator19/4  "RL3 CtrlOutOpt3"
  Demux2/3 -> Bus Creator/3  "FL CtrlOutOpt2"
  Demux4/4 -> Bus Creator2/4  "RL CtrlOutOpt3"
  Demux3/2 -> Bus Creator1/2  "FR CtrlOutOpt1"
  Bus Creator11/1 -> Bus Creator9/5
  Demux2/4 -> Bus Creator/4  "FL CtrlOutOpt3"
  Demux/9 -> Demux18/1  "RL3"
  Demux10/3 -> Bus Creator11/3  "RL2 CtrlOutOpt2"
  Demux2/1 -> Bus Creator/1  "FL CtrlOutOpt0"
  Demux13/4 -> Bus Creator14/4  "FR2 CtrlOutOpt3"
  Demux19/4 -> Bus Creator20/4  "RR3 CtrlOutOpt3"
  Bus Creator1/1 -> Bus Creator9/2
  Bus Creator14/1 -> Bus Creator9/8
  Demux4/3 -> Bus Creator2/3  "RL CtrlOutOpt2"
  Demux2/2 -> Bus Creator/2  "FL CtrlOutOpt1"
  Demux5/1 -> Bus Creator3/1  "RR CtrlOutOpt0"
  Demux18/3 -> Bus Creator19/3  "RL3 CtrlOutOpt2"
  Demux12/1 -> Bus Creator13/1  "FL2 CtrlOutOpt0"
  Demux12/3 -> Bus Creator13/3  "FL2 CtrlOutOpt2"
  Bus Creator19/1 -> Bus Creator9/9
  Demux4/1 -> Bus Creator2/1  "RL CtrlOutOpt0"
  Demux10/1 -> Bus Creator11/1  "RL2 CtrlOutOpt0"
  Bus Creator/1 -> Bus Creator9/1
  Demux11/1 -> Bus Creator12/1  "RR2 CtrlOutOpt0"
  Demux20/1 -> Bus Creator21/1  "RL4 CtrlOutOpt0"
  Demux10/4 -> Bus Creator11/4  "RL2 CtrlOutOpt3"
  Bus Creator12/1 -> Bus Creator9/6
  Demux12/2 -> Bus Creator13/2  "FL2 CtrlOutOpt1"
  Demux11/3 -> Bus Creator12/3  "RR2 CtrlOutOpt2"
  Demux3/4 -> Bus Creator1/4  "FR CtrlOutOpt3"
  Demux18/2 -> Bus Creator19/2  "RL3 CtrlOutOpt1"
  Demux5/3 -> Bus Creator3/3  "RR CtrlOutOpt2"
  Demux19/2 -> Bus Creator20/2  "RR3 CtrlOutOpt1"
  Bus Creator20/1 -> Bus Creator9/10
  Demux20/2 -> Bus Creator21/2  "RL4 CtrlOutOpt1"
  Demux/7 -> Demux12/1  "FL2"
  Bus Creator2/1 -> Bus Creator9/3
  Demux/4 -> Demux5/1  "RR"
  Demux/1 -> Demux2/1  "FL"
  Demux20/4 -> Bus Creator21/4  "RL4 CtrlOutOpt3"
  Demux13/1 -> Bus Creator14/1  "FR2 CtrlOutOpt0"
  Demux/3 -> Demux4/1  "RL"
  Demux20/3 -> Bus Creator21/3  "RL4 CtrlOutOpt2"
  Demux3/1 -> Bus Creator1/1  "FR CtrlOutOpt0"
  Demux21/4 -> Bus Creator22/4  "RR4 CtrlOutOpt3"
  Demux11/4 -> Bus Creator12/4  "RR2 CtrlOutOpt3"
  Demux3/3 -> Bus Creator1/3  "FR CtrlOutOpt2"
  Demux18/1 -> Bus Creator19/1  "RL3 CtrlOutOpt0"
  Demux/10 -> Demux19/1  "RR3"
  Demux10/2 -> Bus Creator11/2  "RL2 CtrlOutOpt1"
  Demux12/4 -> Bus Creator13/4  "FL2 CtrlOutOpt3"
  Demux13/3 -> Bus Creator14/3  "FR2 CtrlOutOpt2"
  Demux4/2 -> Bus Creator2/2  "RL CtrlOutOpt1"
  Demux21/2 -> Bus Creator22/2  "RR4 CtrlOutOpt1"
  Demux5/2 -> Bus Creator3/2  "RR CtrlOutOpt1"
  Bus Creator3/1 -> Bus Creator9/4
  Demux21/3 -> Bus Creator22/3  "RR4 CtrlOutOpt2"
  Demux21/1 -> Bus Creator22/1  "RR4 CtrlOutOpt0"
  Demux/6 -> Demux11/1  "RR2"
  Demux/2 -> Demux3/1  "FR"
  Demux11/2 -> Bus Creator12/2  "RR2 CtrlOutOpt1"
  Demux13/2 -> Bus Creator14/2  "FR2 CtrlOutOpt1"
  Demux/5 -> Demux10/1  "RL2"
  Bus Creator13/1 -> Bus Creator9/7
  Demux5/4 -> Bus Creator3/4  "RR CtrlOutOpt3"
  In/1 -> Demux/1
  Bus Creator9/1 -> Out/1
  Demux/11 -> Demux20/1  "RL4"
  Bus Creator21/1 -> Bus Creator9/11
  Demux/12 -> Demux21/1  "RR4"
  Bus Creator22/1 -> Bus Creator9/12

== system generic_Truck_And_Trailer/TruckMaker/IPG Vehicle/CarAndTrailer/Forces/Suspension Forces/CreateBus BufferCtrlOutOpt ==
  note: <Your model here>
  In : Inport
  Bus Creator{,1..3,11..14,19..22} (12 alike) : BusCreator  Inputs=4
  Bus Creator9 : BusCreator  Inputs=12
  Demux : Demux  Outputs=12
  Demux{2..5,10..13,18..21} (12 alike) : Demux
  Out : Outport
  wires:
  Demux/8 -> Demux13/1  "FR2"
  Demux19/1 -> Bus Creator20/1  "RR3 CtrlOutOpt0"
  Demux19/3 -> Bus Creator20/3  "RR3 CtrlOutOpt2"
  Demux18/4 -> Bus Creator19/4  "RL3 CtrlOutOpt3"
  Demux2/3 -> Bus Creator/3  "FL CtrlOutOpt2"
  Demux4/4 -> Bus Creator2/4  "RL CtrlOutOpt3"
  Demux3/2 -> Bus Creator1/2  "FR CtrlOutOpt1"
  Bus Creator11/1 -> Bus Creator9/5
  Demux2/4 -> Bus Creator/4  "FL CtrlOutOpt3"
  Demux/9 -> Demux18/1  "RL3"
  Demux10/3 -> Bus Creator11/3  "RL2 CtrlOutOpt2"
  Demux2/1 -> Bus Creator/1  "FL CtrlOutOpt0"
  Demux13/4 -> Bus Creator14/4  "FR2 CtrlOutOpt3"
  Demux19/4 -> Bus Creator20/4  "RR3 CtrlOutOpt3"
  Bus Creator1/1 -> Bus Creator9/2
  Bus Creator14/1 -> Bus Creator9/8
  Demux4/3 -> Bus Creator2/3  "RL CtrlOutOpt2"
  Demux2/2 -> Bus Creator/2  "FL CtrlOutOpt1"
  Demux5/1 -> Bus Creator3/1  "RR CtrlOutOpt0"
  Demux18/3 -> Bus Creator19/3  "RL3 CtrlOutOpt2"
  Demux12/1 -> Bus Creator13/1  "FL2 CtrlOutOpt0"
  Demux12/3 -> Bus Creator13/3  "FL2 CtrlOutOpt2"
  Bus Creator19/1 -> Bus Creator9/9
  Demux4/1 -> Bus Creator2/1  "RL CtrlOutOpt0"
  Demux10/1 -> Bus Creator11/1  "RL2 CtrlOutOpt0"
  Bus Creator/1 -> Bus Creator9/1
  Demux11/1 -> Bus Creator12/1  "RR2 CtrlOutOpt0"
  Demux20/1 -> Bus Creator21/1  "RL4 CtrlOutOpt0"
  Demux10/4 -> Bus Creator11/4  "RL2 CtrlOutOpt3"
  Bus Creator12/1 -> Bus Creator9/6
  Demux12/2 -> Bus Creator13/2  "FL2 CtrlOutOpt1"
  Demux11/3 -> Bus Creator12/3  "RR2 CtrlOutOpt2"
  Demux3/4 -> Bus Creator1/4  "FR CtrlOutOpt3"
  Demux18/2 -> Bus Creator19/2  "RL3 CtrlOutOpt1"
  Demux5/3 -> Bus Creator3/3  "RR CtrlOutOpt2"
  Demux19/2 -> Bus Creator20/2  "RR3 CtrlOutOpt1"
  Bus Creator20/1 -> Bus Creator9/10
  Demux20/2 -> Bus Creator21/2  "RL4 CtrlOutOpt1"
  Demux/7 -> Demux12/1  "FL2"
  Bus Creator2/1 -> Bus Creator9/3
  Demux/4 -> Demux5/1  "RR"
  Demux/1 -> Demux2/1  "FL"
  Demux20/4 -> Bus Creator21/4  "RL4 CtrlOutOpt3"
  Demux13/1 -> Bus Creator14/1  "FR2 CtrlOutOpt0"
  Demux/3 -> Demux4/1  "RL"
  Demux20/3 -> Bus Creator21/3  "RL4 CtrlOutOpt2"
  Demux3/1 -> Bus Creator1/1  "FR CtrlOutOpt0"
  Demux21/4 -> Bus Creator22/4  "RR4 CtrlOutOpt3"
  Demux11/4 -> Bus Creator12/4  "RR2 CtrlOutOpt3"
  Demux3/3 -> Bus Creator1/3  "FR CtrlOutOpt2"
  Demux18/1 -> Bus Creator19/1  "RL3 CtrlOutOpt0"
  Demux/10 -> Demux19/1  "RR3"
  Demux10/2 -> Bus Creator11/2  "RL2 CtrlOutOpt1"
  Demux12/4 -> Bus Creator13/4  "FL2 CtrlOutOpt3"
  Demux13/3 -> Bus Creator14/3  "FR2 CtrlOutOpt2"
  Demux4/2 -> Bus Creator2/2  "RL CtrlOutOpt1"
  Demux21/2 -> Bus Creator22/2  "RR4 CtrlOutOpt1"
  Demux5/2 -> Bus Creator3/2  "RR CtrlOutOpt1"
  Bus Creator3/1 -> Bus Creator9/4
  Demux21/3 -> Bus Creator22/3  "RR4 CtrlOutOpt2"
  Demux21/1 -> Bus Creator22/1  "RR4 CtrlOutOpt0"
  Demux/6 -> Demux11/1  "RR2"
  Demux/2 -> Demux3/1  "FR"
  Demux11/2 -> Bus Creator12/2  "RR2 CtrlOutOpt1"
  Demux13/2 -> Bus Creator14/2  "FR2 CtrlOutOpt1"
  Demux/5 -> Demux10/1  "RL2"
  Bus Creator13/1 -> Bus Creator9/7
  Demux5/4 -> Bus Creator3/4  "RR CtrlOutOpt3"
  In/1 -> Demux/1
  Bus Creator9/1 -> Out/1
  Demux/11 -> Demux20/1  "RL4"
  Bus Creator21/1 -> Bus Creator9/11
  Demux/12 -> Demux21/1  "RR4"
  Bus Creator22/1 -> Bus Creator9/12

== system generic_Truck_And_Trailer/TruckMaker/IPG Vehicle/CarAndTrailer/Forces/Suspension Forces/CreateBus DamperCtrlOutOpt ==
  note: <Your model here>
  In : Inport
  Bus Creator{,1..3,11..14,19..22} (12 alike) : BusCreator  Inputs=4
  Bus Creator9 : BusCreator  Inputs=12
  Demux : Demux  Outputs=12
  Demux{2..5,10..13,18..21} (12 alike) : Demux
  Out : Outport
  wires:
  Demux/8 -> Demux13/1  "FR2"
  Demux19/1 -> Bus Creator20/1  "RR3 CtrlOutOpt0"
  Demux19/3 -> Bus Creator20/3  "RR3 CtrlOutOpt2"
  Demux18/4 -> Bus Creator19/4  "RL3 CtrlOutOpt3"
  Demux2/3 -> Bus Creator/3  "FL CtrlOutOpt2"
  Demux4/4 -> Bus Creator2/4  "RL CtrlOutOpt3"
  Demux3/2 -> Bus Creator1/2  "FR CtrlOutOpt1"
  Bus Creator11/1 -> Bus Creator9/5
  Demux2/4 -> Bus Creator/4  "FL CtrlOutOpt3"
  Demux/9 -> Demux18/1  "RL3"
  Demux10/3 -> Bus Creator11/3  "RL2 CtrlOutOpt2"
  Demux2/1 -> Bus Creator/1  "FL CtrlOutOpt0"
  Demux13/4 -> Bus Creator14/4  "FR2 CtrlOutOpt3"
  Demux19/4 -> Bus Creator20/4  "RR3 CtrlOutOpt3"
  Bus Creator1/1 -> Bus Creator9/2
  Bus Creator14/1 -> Bus Creator9/8
  Demux4/3 -> Bus Creator2/3  "RL CtrlOutOpt2"
  Demux2/2 -> Bus Creator/2  "FL CtrlOutOpt1"
  Demux5/1 -> Bus Creator3/1  "RR CtrlOutOpt0"
  Demux18/3 -> Bus Creator19/3  "RL3 CtrlOutOpt2"
  Demux12/1 -> Bus Creator13/1  "FL2 CtrlOutOpt0"
  Demux12/3 -> Bus Creator13/3  "FL2 CtrlOutOpt2"
  Bus Creator19/1 -> Bus Creator9/9
  Demux4/1 -> Bus Creator2/1  "RL CtrlOutOpt0"
  Demux10/1 -> Bus Creator11/1  "RL2 CtrlOutOpt0"
  Bus Creator/1 -> Bus Creator9/1
  Demux11/1 -> Bus Creator12/1  "RR2 CtrlOutOpt0"
  Demux20/1 -> Bus Creator21/1  "RL4 CtrlOutOpt0"
  Demux10/4 -> Bus Creator11/4  "RL2 CtrlOutOpt3"
  Bus Creator12/1 -> Bus Creator9/6
  Demux12/2 -> Bus Creator13/2  "FL2 CtrlOutOpt1"
  Demux11/3 -> Bus Creator12/3  "RR2 CtrlOutOpt2"
  Demux3/4 -> Bus Creator1/4  "FR CtrlOutOpt3"
  Demux18/2 -> Bus Creator19/2  "RL3 CtrlOutOpt1"
  Demux5/3 -> Bus Creator3/3  "RR CtrlOutOpt2"
  Demux19/2 -> Bus Creator20/2  "RR3 CtrlOutOpt1"
  Bus Creator20/1 -> Bus Creator9/10
  Demux20/2 -> Bus Creator21/2  "RL4 CtrlOutOpt1"
  Demux/7 -> Demux12/1  "FL2"
  Bus Creator2/1 -> Bus Creator9/3
  Demux/4 -> Demux5/1  "RR"
  Demux/1 -> Demux2/1  "FL"
  Demux20/4 -> Bus Creator21/4  "RL4 CtrlOutOpt3"
  Demux13/1 -> Bus Creator14/1  "FR2 CtrlOutOpt0"
  Demux/3 -> Demux4/1  "RL"
  Demux20/3 -> Bus Creator21/3  "RL4 CtrlOutOpt2"
  Demux3/1 -> Bus Creator1/1  "FR CtrlOutOpt0"
  Demux21/4 -> Bus Creator22/4  "RR4 CtrlOutOpt3"
  Demux11/4 -> Bus Creator12/4  "RR2 CtrlOutOpt3"
  Demux3/3 -> Bus Creator1/3  "FR CtrlOutOpt2"
  Demux18/1 -> Bus Creator19/1  "RL3 CtrlOutOpt0"
  Demux/10 -> Demux19/1  "RR3"
  Demux10/2 -> Bus Creator11/2  "RL2 CtrlOutOpt1"
  Demux12/4 -> Bus Creator13/4  "FL2 CtrlOutOpt3"
  Demux13/3 -> Bus Creator14/3  "FR2 CtrlOutOpt2"
  Demux4/2 -> Bus Creator2/2  "RL CtrlOutOpt1"
  Demux21/2 -> Bus Creator22/2  "RR4 CtrlOutOpt1"
  Demux5/2 -> Bus Creator3/2  "RR CtrlOutOpt1"
  Bus Creator3/1 -> Bus Creator9/4
  Demux21/3 -> Bus Creator22/3  "RR4 CtrlOutOpt2"
  Demux21/1 -> Bus Creator22/1  "RR4 CtrlOutOpt0"
  Demux/6 -> Demux11/1  "RR2"
  Demux/2 -> Demux3/1  "FR"
  Demux11/2 -> Bus Creator12/2  "RR2 CtrlOutOpt1"
  Demux13/2 -> Bus Creator14/2  "FR2 CtrlOutOpt1"
  Demux/5 -> Demux10/1  "RL2"
  Bus Creator13/1 -> Bus Creator9/7
  Demux5/4 -> Bus Creator3/4  "RR CtrlOutOpt3"
  In/1 -> Demux/1
  Bus Creator9/1 -> Out/1
  Demux/11 -> Demux20/1  "RL4"
  Bus Creator21/1 -> Bus Creator9/11
  Demux/12 -> Demux21/1  "RR4"
  Bus Creator22/1 -> Bus Creator9/12
